simulink model "sistema"  (R2015b)
settings: Solver=VariableStepAuto  StartTime=0.0  StopTime=Tt  RelTol=1e-3
undefined symbols (not defined in the file): a, A, Ad, b, B, Bd, c, C, Cd, D, Dd, Ts, x1, x2, x3, x4
settings Model: Creator=pdoren  LastModifiedBy=pdoren

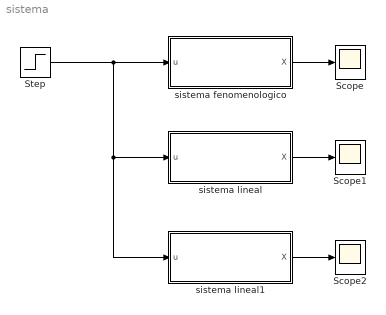
== system sistema ==
  Scope : Scope
  Scope1 : Scope
  Scope2 : Scope
  Step : Step  After=0  SampleTime=0
  sistema fenomenologico : Subsystem
  sistema lineal : Subsystem
  sistema lineal1 : Subsystem
  wires:
  sistema fenomenologico/1(X) -> Scope/1
  sistema lineal/1(X) -> Scope1/1
  Step/1 -> sistema lineal1/1(u), sistema lineal/1(u), sistema fenomenologico/1(u)
  sistema lineal1/1(X) -> Scope2/1

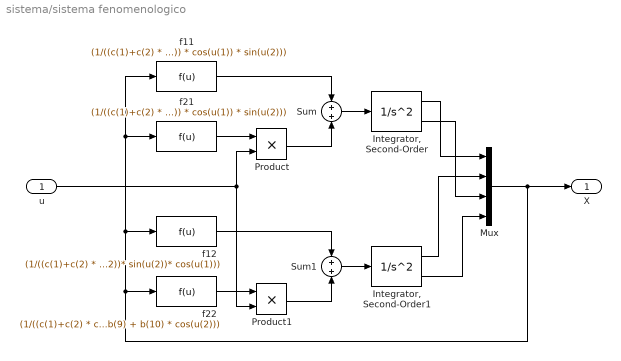
== system sistema/sistema fenomenologico ==
  u : Inport
  "Integrator, Second-Order" : SecondOrderIntegrator  ICX=x1  ICDXDT=x3
  "Integrator, Second-Order1" : SecondOrderIntegrator  ICX=x2  ICDXDT=x4
  Mux : Mux
  Product : Product
  Product1 : Product
  Sum : Sum  Inputs=+|+
  Sum1 : Sum  Inputs=+|+
  f11 : Fcn  Expr=(1/((c(1)+c(2) * cos(u(2))^2) * c(3))) * ((a(1) + a(2) * cos(u(2))) * sin(u(2)) * u(3)^2 + a(3) * sin(u(2)) * u(4) * u(3) + a(4) * sin(u(2)) * u(4)^2 + (a(5) + a(6) * cos(u(2))) * u(4) + a(9) * sin(u(1)) * cos(u(2))^2 + a(10) * sin(u(1)) + a(11) * cos(u(2)) * cos(u(1)) * sin(u(2)))
  f12 : Fcn  Expr=(1/((c(1)+c(2) * cos(u(2))^2) * c(3))) * ((b(1) + b(2) * cos(u(2))) * sin(u(2)) * u(3)^2 + (b(3) * cos(u(2)) + b(4))* sin(u(2)) * u(4) * u(1) + (b(5) + b(6) * cos(u(2)))* sin(u(2)) * u(4)^2 + (b(7) + b(8)* cos(u(2))) * u(4) + (b(11) + b(12)* cos(u(2)))* sin(u(1)) + b(13) * sin(u(1)) * cos(u(2))^2 + b(14) * cos(u(1)) * sin(u(2)) + b(15) * cos(u(2))* sin(u(2))* cos(u(1)))
  f21 : Fcn  Expr=(1/((c(1)+c(2) * cos(u(2))^2) * c(3))) * ((a(1) + a(2) * cos(u(2))) * sin(u(2)) * u(3)^2 + a(3) * sin(u(2)) * u(4) * u(3) + a(4) * sin(u(2)) * u(4)^2 + (a(5) + a(6) * cos(u(2))) * u(4) + a(9) * sin(u(1)) * cos(u(2))^2 + a(10) * sin(u(1)) + a(11) * cos(u(2)) * cos(u(1)) * sin(u(2)))
  f22 : Fcn  Expr=(1/((c(1)+c(2) * cos(u(2))^2) * c(3))) * (b(9) + b(10) * cos(u(2)))
  X : Outport
  wires:
  Product/1 -> Sum/2
  f11/1 -> Sum/1
  f21/1 -> Product/1
  "Integrator, Second-Order"/1 -> Mux/1
  "Integrator, Second-Order1"/2 -> Mux/4
  Sum1/1 -> "Integrator, Second-Order1"/1
  "Integrator, Second-Order"/2 -> Mux/3
  "Integrator, Second-Order1"/1 -> Mux/2
  u/1 -> Product1/2, Product/2
  Mux/1 -> X/1, f22/1, f12/1, f21/1, f11/1
  Sum/1 -> "Integrator, Second-Order"/1
  f12/1 -> Sum1/1
  f22/1 -> Product1/1
  Product1/1 -> Sum1/2

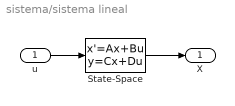
== system sistema/sistema lineal ==
  u : Inport
  State-Space : StateSpace  A=A  B=B  C=C  D=D  X0=[x1 x2 x3 x4]
  X : Outport
  wires:
  u/1 -> State-Space/1
  State-Space/1 -> X/1

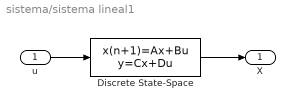
== system sistema/sistema lineal1 ==
  u : Inport
  Discrete State-Space : DiscreteStateSpace  A=Ad  B=Bd  C=Cd  D=Dd  X0=[x1 x2 x3 x4]  SampleTime=Ts
  X : Outport
  wires:
  u/1 -> Discrete State-Space/1
  Discrete State-Space/1 -> X/1
